simulink model "Retroacao_de_estados_1a_Lei_simulink"  (R2019a)
settings: Solver=ode45  StartTime=0.0  StopTime=4  RelTol=1e-3  EnableMultiTasking=on
values from neighbouring files (symbols this model uses):
  a = [-1 1; 1 -2]    [Ganhos_observador_de_estados.m]    (also in Observador_de_estados.m; Retroacao_de_estados_1a_Lei.m = [0 1; -40 -3]; Retroacao_de_estados_2a_Lei.m = [[0 1]; [0 -50]])
  b = [1;0]    [Ganhos_observador_de_estados.m]    (also in Observador_de_estados.m; Retroacao_de_estados_1a_Lei.m = [0 ; 40]; Retroacao_de_estados_2a_Lei.m = [0;1370])
  K1 = K(1)    [Retroacao_de_estados_1a_Lei.m]    (also in Retroacao_de_estados_2a_Lei.m; Retroacao_de_estados_3a_Lei.m)
  K2 = K(2)    [Retroacao_de_estados_1a_Lei.m]    (also in Retroacao_de_estados_2a_Lei.m)
  x1_ini = 0.05    [Retroacao_de_estados_1a_Lei.m]
  x2_ini = 0.05    [Retroacao_de_estados_1a_Lei.m]
settings Model: Creator=Joao Paulo  LastModifiedBy=mathe
settings DataIOCC: LimitDataPoints=on  SaveFormat=Array  ReturnWorkspaceOutputs=off
settings OptimizationCC: ExpressionDepthLimit=2147483647  LifeSpan=inf
settings DebuggingCC: UnderspecifiedInitializationDetection=Classic  MergeDetectMultiDrivingBlocksExec=none  SolverPrmCheckMsg=warning  StateNameClashWarn=warning  SFUnexpectedBacktrackingDiag=warning  SFNoUnconditionalDefaultTransitionDiag=warning  SFExecutionAtInitializationDiag=none  ArithmeticOperatorsInVariantConditions=warning
settings HardwareCC: ProdBitPerPointer=32  ProdBitPerSizeT=32  ProdBitPerPtrDiffT=32  ProdLargestAtomicFloat=None  ProdIntDivRoundTo=Undefined  ProdEndianess=Unspecified  ProdWordSize=32  ProdHWDeviceType=32-bit Generic
settings ModelReferenceCC: PropagateSignalLabelsOutOfModel=off
settings SFSimCC: SimUseLocalCustomCode=off
settings RTWCC: RTWUseLocalCustomCode=off
settings CodeAppCC: StateflowObjectComments=on
settings GRTTargetCC: TargetLangStandard=C89/C90 (ANSI)  GeneratePreprocessorConditionals=Disable all
settings ConfigComp: CovMetricSettings=dw  CovHtmlReporting=on  CovSaveCumulativeToWorkspaceVar=on  CovSaveSingleToWorkspaceVar=on  CovExternalEMLEnable=off

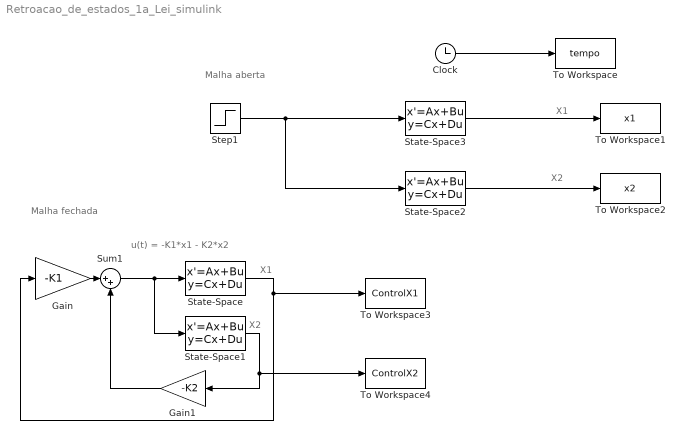
== system Retroacao_de_estados_1a_Lei_simulink ==
  note: Malha fechada
  note: Malha aberta
  note: u(t) = -K1*x1 - K2*x2
  note: X2
  note: X1
  note: X2
  note: X1
  Clock : Clock
  Gain : Gain  Gain=-K1
  Gain1 : Gain  Gain=-K2
  State-Space : StateSpace  A=a  B=b  C=[1 0]  D=0  InitialCondition=x1_ini
  State-Space1 : StateSpace  A=a  B=b  C=[0 1]  D=0  InitialCondition=x2_ini
  State-Space2 : StateSpace  A=a  B=b  C=[0 1]  D=0  InitialCondition=0.05
  State-Space3 : StateSpace  A=a  B=b  C=[1 0]  D=0  InitialCondition=0.05
  Step1 : Step  Time=0  After=0  SampleTime=0
  Sum1 : Sum  Inputs=|++
  To Workspace : ToWorkspace  VariableName=tempo  SampleTime=-1
  To Workspace1 : ToWorkspace  VariableName=x1  SampleTime=-1
  To Workspace2 : ToWorkspace  VariableName=x2  SampleTime=-1
  To Workspace3 : ToWorkspace  VariableName=ControlX1  SampleTime=-1
  To Workspace4 : ToWorkspace  VariableName=ControlX2  SampleTime=-1
  wires:
  Clock/1 -> To Workspace/1
  Gain/1 -> Sum1/1
  Sum1/1 -> State-Space1/1, State-Space/1
  State-Space1/1 -> Gain1/1, To Workspace4/1
  State-Space/1 -> To Workspace3/1, Gain/1
  Gain1/1 -> Sum1/2
  Step1/1 -> State-Space2/1, State-Space3/1
  State-Space3/1 -> To Workspace1/1
  State-Space2/1 -> To Workspace2/1
